simulink model "Assignment_2"  (R2022a)
settings: Solver=FixedStepAuto  StartTime=0.0  StopTime=10  FixedStep=1e-3  RelTol=1e-3  EnableMultiTasking=on
undefined symbols (not defined in the file or in its folder): D0, D1, D10, D11, D12, D13, D2, D3, D4, D5, D6, D7, D8, D9, PTA0, PTA1, PTA2, PTB23, PTB9, PTC16, PTC17, PTC2, PTC3, PTC4, PTD0, PTD1, PTD2, PTD3
libraries: etargetslib x25, frdmk64flib x16
settings Model: ExtModeTrigDuration=5  Creator=anand  LastModifiedBy=anand
settings DataIOCC: ReturnWorkspaceOutputs=off
settings OptimizationCC: EnhancedBackFolding=on  PassReuseOutputArgsAs=Individual arguments  ZeroExternalMemoryAtStartup=off  ZeroInternalMemoryAtStartup=off  MaxStackSize=64  OptimizeBlockOrder=speed  DifferentSizesBufferReuse=on  OptimizationCustomize=off  EfficientTunableParamExpr=on
settings DebuggingCC: ParameterTunabilityLossMsg=error
settings HardwareCC: ProdBitPerPointer=32  ProdBitPerSizeT=32  ProdBitPerPtrDiffT=32  ProdLargestAtomicInteger=Long  ProdLargestAtomicFloat=Double  ProdWordSize=32  ProdHWDeviceType=ARM Compatible->ARM Cortex
settings SFSimCC: MATLABDynamicMemAlloc=off
settings RTWCC: SystemTargetFile=ert.tlc  HardwareBoard=NXP FRDM-K64F  TLCOptions="-aInlineSetEventsForThisBaseRateFcn=TLC_FALSE -aSuppressMultiTaskScheduler=TLC_FALSE  -aRateBasedStepFcn=0"  TemplateMakefile=ert_default_tmf  Toolchain=GNU Tools for ARM Embedded Processors
settings CodeAppCC: ForceParamTrailComments=on  IgnoreCustomStorageClasses=off  OperatorAnnotations=on  SimulinkDataObjDesc=on  SFDataObjDesc=on  InsertBlockDesc=on
settings ERTTargetCC: ExtModeTransport=4  ExtModeMexFile=sendToCommService

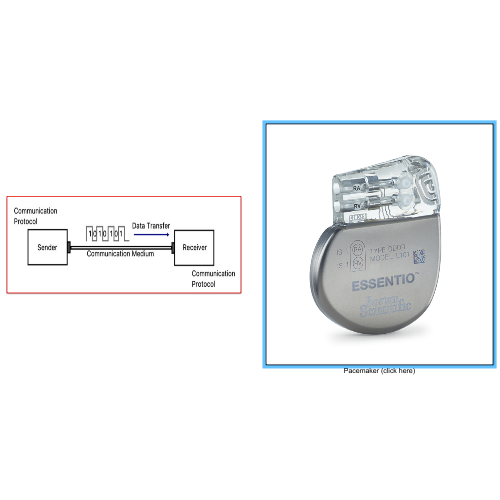
[thumbnail: Simulink's stored preview of the top-level diagram]
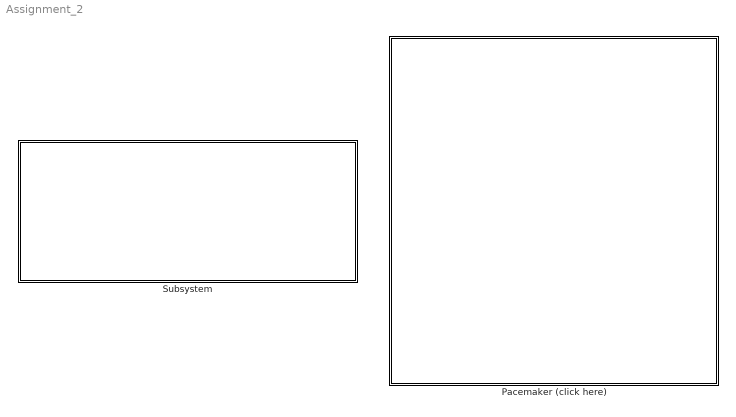
== system Assignment_2 ==
  Pacemaker (click here) : Subsystem
      mask Display: image('$imagefile'); % Use "Edit Image" on toolstrip to change.
  Subsystem : Subsystem
      mask Display: image('C:\Users\anand\Desktop\Screenshot 2022-11-24 140132.jpg'); % Use "Edit Image" on toolstrip to change.

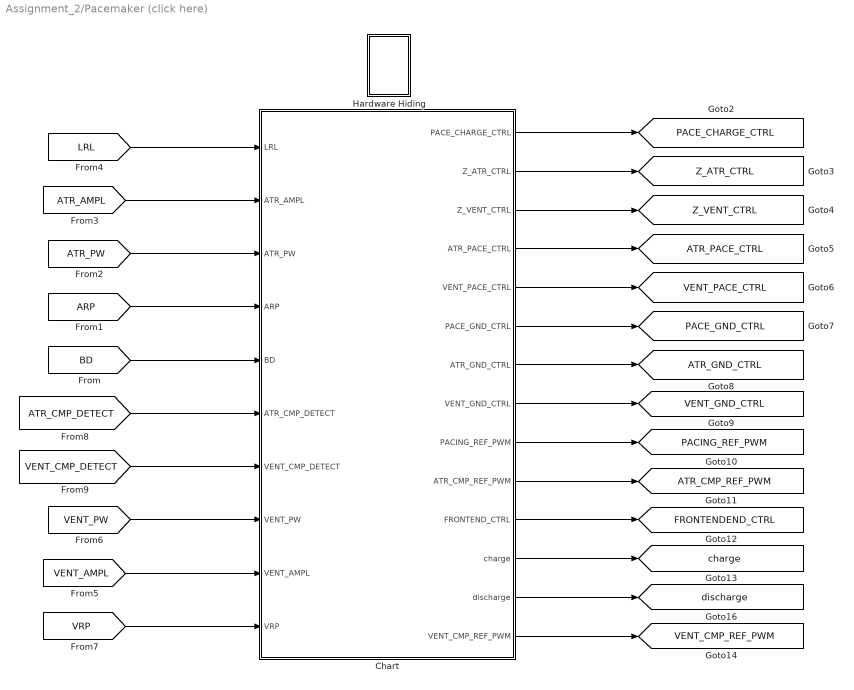
== system Assignment_2/Pacemaker (click here) ==
  Chart : Stateflow chart  TreatAsAtomicUnit=on
  Hardware Hiding : Subsystem
  tag scope: ATR_CMP_REF_PWM=global, ATR_GND_CTRL=global, ATR_PACE_CTRL=global, FRONTENDEND_CTRL=global, PACE_CHARGE_CTRL=global, PACE_GND_CTRL=global, PACING_REF_PWM=global, VENT_CMP_REF_PWM=global, VENT_GND_CTRL=global, VENT_PACE_CTRL=global, Z_ATR_CTRL=global, Z_VENT_CTRL=global, charge=global, discharge=global
  wires:
  Chart/9(PACING_REF_PWM) -> [PACING_REF_PWM]
  Chart/11(FRONTEND_CTRL) -> [FRONTENDEND_CTRL]
  Chart/10(ATR_CMP_REF_PWM) -> [ATR_CMP_REF_PWM]
  [ATR_CMP_DETECT] -> Chart/6(ATR_CMP_DETECT)
  [LRL] -> Chart/1(LRL)
  [VENT_AMPL] -> Chart/9(VENT_AMPL)
  Chart/4(ATR_PACE_CTRL) -> [ATR_PACE_CTRL]
  [ARP] -> Chart/4(ARP)
  [ATR_PW] -> Chart/3(ATR_PW)
  [BD] -> Chart/5(BD)
  Chart/14(VENT_CMP_REF_PWM) -> [VENT_CMP_REF_PWM]
  Chart/5(VENT_PACE_CTRL) -> [VENT_PACE_CTRL]
  Chart/12(charge) -> [charge]
  [ATR_AMPL] -> Chart/2(ATR_AMPL)
  Chart/6(PACE_GND_CTRL) -> [PACE_GND_CTRL]
  Chart/13(discharge) -> [discharge]
  Chart/2(Z_ATR_CTRL) -> [Z_ATR_CTRL]
  [VRP] -> Chart/10(VRP)
  Chart/3(Z_VENT_CTRL) -> [Z_VENT_CTRL]
  [VENT_CMP_DETECT] -> Chart/7(VENT_CMP_DETECT)
  Chart/7(ATR_GND_CTRL) -> [ATR_GND_CTRL]
  Chart/8(VENT_GND_CTRL) -> [VENT_GND_CTRL]
  Chart/1(PACE_CHARGE_CTRL) -> [PACE_CHARGE_CTRL]
  [VENT_PW] -> Chart/8(VENT_PW)

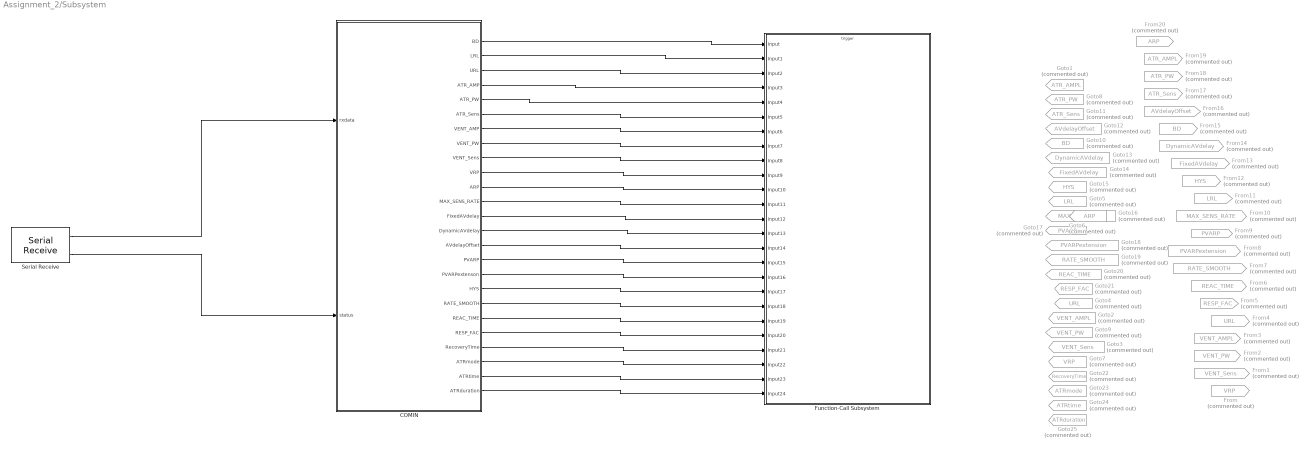
== system Assignment_2/Subsystem ==
  COMIN : Stateflow chart  TreatAsAtomicUnit=on
  From : From  Commented=on  GotoTag=VRP  TagVisibility=global
  From1 : From  Commented=on  GotoTag=VENT_Sens  TagVisibility=global
  From10 : From  Commented=on  GotoTag=MAX_SENS_RATE  TagVisibility=global
  From11 : From  Commented=on  GotoTag=LRL  TagVisibility=global
  From12 : From  Commented=on  GotoTag=HYS  TagVisibility=global
  From13 : From  Commented=on  GotoTag=FixedAVdelay  TagVisibility=global
  From14 : From  Commented=on  GotoTag=DynamicAVdelay  TagVisibility=global
  From15 : From  Commented=on  GotoTag=BD  TagVisibility=global
  From16 : From  Commented=on  GotoTag=AVdelayOffset  TagVisibility=global
  From17 : From  Commented=on  GotoTag=ATR_Sens  TagVisibility=global
  From18 : From  Commented=on  GotoTag=ATR_PW  TagVisibility=global
  From19 : From  Commented=on  GotoTag=ATR_AMPL  TagVisibility=global
  From2 : From  Commented=on  GotoTag=VENT_PW  TagVisibility=global
  From20 : From  Commented=on  GotoTag=ARP  TagVisibility=global
  From3 : From  Commented=on  GotoTag=VENT_AMPL  TagVisibility=global
  From4 : From  Commented=on  GotoTag=URL  TagVisibility=global
  From5 : From  Commented=on  GotoTag=RESP_FAC  TagVisibility=global
  From6 : From  Commented=on  GotoTag=REAC_TIME  TagVisibility=global
  From7 : From  Commented=on  GotoTag=RATE_SMOOTH  TagVisibility=global
  From8 : From  Commented=on  GotoTag=PVARPextension  TagVisibility=global
  From9 : From  Commented=on  GotoTag=PVARP  TagVisibility=global
  Function-Call Subsystem : Subsystem  TreatAsAtomicUnit=on
  Goto1 : Goto  Commented=on  GotoTag=ATR_AMPL  TagVisibility=global
  Goto10 : Goto  Commented=on  GotoTag=BD  TagVisibility=global
  Goto11 : Goto  Commented=on  GotoTag=ATR_Sens  TagVisibility=global
  Goto12 : Goto  Commented=on  GotoTag=AVdelayOffset  TagVisibility=global
  Goto13 : Goto  Commented=on  GotoTag=DynamicAVdelay  TagVisibility=global
  Goto14 : Goto  Commented=on  GotoTag=FixedAVdelay  TagVisibility=global
  Goto15 : Goto  Commented=on  GotoTag=HYS  TagVisibility=global
  Goto16 : Goto  Commented=on  GotoTag=MAX_SENS_RATE  TagVisibility=global
  Goto17 : Goto  Commented=on  GotoTag=PVARP  TagVisibility=global
  Goto18 : Goto  Commented=on  GotoTag=PVARPextension  TagVisibility=global
  Goto19 : Goto  Commented=on  GotoTag=RATE_SMOOTH  TagVisibility=global
  Goto2 : Goto  Commented=on  GotoTag=VENT_AMPL  TagVisibility=global
  Goto20 : Goto  Commented=on  GotoTag=REAC_TIME  TagVisibility=global
  Goto21 : Goto  Commented=on  GotoTag=RESP_FAC  TagVisibility=global
  Goto22 : Goto  Commented=on  GotoTag=RecoveryTime  TagVisibility=global
  Goto23 : Goto  Commented=on  GotoTag=ATRmode  TagVisibility=global
  Goto24 : Goto  Commented=on  GotoTag=ATRtime  TagVisibility=global
  Goto25 : Goto  Commented=on  GotoTag=ATRduration  TagVisibility=global
  Goto3 : Goto  Commented=on  GotoTag=VENT_Sens  TagVisibility=global
  Goto4 : Goto  Commented=on  GotoTag=URL  TagVisibility=global
  Goto5 : Goto  Commented=on  GotoTag=LRL  TagVisibility=global
  Goto6 : Goto  Commented=on  GotoTag=ARP  TagVisibility=global
  Goto7 : Goto  Commented=on  GotoTag=VRP  TagVisibility=global
  Goto8 : Goto  Commented=on  GotoTag=ATR_PW  TagVisibility=global
  Goto9 : Goto  Commented=on  GotoTag=VENT_PW  TagVisibility=global
  Serial Receive : frdmk64flib/Serial Receive  SCIModule=0  Baudrate=uint32(9600)  Parity=None  StopBits=1  HardwareFlowControl=None  ByteOrder=LittleEndian  DataType=uint8  DataLength=101  BlockingMode=off  OutputStatus=on  SampleTime=-1
  wires:
  Serial Receive/1 -> COMIN/1(rxdata)
  Serial Receive/2 -> COMIN/2(status)
  COMIN/1(BD) -> Function-Call Subsystem/1(Input)
  COMIN/2(LRL) -> Function-Call Subsystem/2(Input1)
  COMIN/3(URL) -> Function-Call Subsystem/3(Input2)
  COMIN/4(ATR_AMP) -> Function-Call Subsystem/4(Input3)
  COMIN/5(ATR_PW) -> Function-Call Subsystem/5(Input4)
  COMIN/6(ATR_Sens) -> Function-Call Subsystem/6(Input5)
  COMIN/7(VENT_AMP) -> Function-Call Subsystem/7(Input6)
  COMIN/8(VENT_PW) -> Function-Call Subsystem/8(Input7)
  COMIN/9(VENT_Sens) -> Function-Call Subsystem/9(Input8)
  COMIN/10(VRP) -> Function-Call Subsystem/10(Input9)
  COMIN/11(ARP) -> Function-Call Subsystem/11(Input10)
  COMIN/12(MAX_SENS_RATE) -> Function-Call Subsystem/12(Input11)
  COMIN/13(FixedAVdelay) -> Function-Call Subsystem/13(Input12)
  COMIN/14(DynamicAVdelay) -> Function-Call Subsystem/14(Input13)
  COMIN/15(AVdelayOffset) -> Function-Call Subsystem/15(Input14)
  COMIN/16(PVARP) -> Function-Call Subsystem/16(Input15)
  COMIN/17(PVARPextenson) -> Function-Call Subsystem/17(Input16)
  COMIN/18(HYS) -> Function-Call Subsystem/18(Input17)
  COMIN/19(RATE_SMOOTH) -> Function-Call Subsystem/19(Input18)
  COMIN/20(REAC_TIME) -> Function-Call Subsystem/20(Input19)
  COMIN/21(RESP_FAC) -> Function-Call Subsystem/21(Input20)
  COMIN/22(RecoveryTime) -> Function-Call Subsystem/22(Input21)
  COMIN/23(ATRmode) -> Function-Call Subsystem/23(Input22)
  COMIN/24(ATRtime) -> Function-Call Subsystem/24(Input23)
  COMIN/25(ATRduration) -> Function-Call Subsystem/25(Input24)

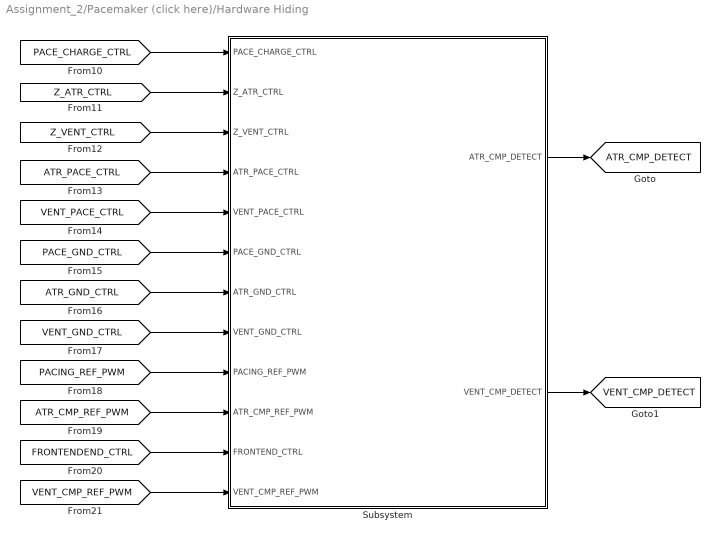
== system Assignment_2/Pacemaker (click here)/Hardware Hiding ==
  Subsystem : Subsystem
  tag scope: ATR_CMP_DETECT=global, VENT_CMP_DETECT=global
  wires:
  [PACE_GND_CTRL] -> Subsystem/6(PACE_GND_CTRL)
  Subsystem/1(ATR_CMP_DETECT) -> [ATR_CMP_DETECT]
  [Z_ATR_CTRL] -> Subsystem/2(Z_ATR_CTRL)
  [FRONTENDEND_CTRL] -> Subsystem/11(FRONTEND_CTRL)
  [ATR_CMP_REF_PWM] -> Subsystem/10(ATR_CMP_REF_PWM)
  [Z_VENT_CTRL] -> Subsystem/3(Z_VENT_CTRL)
  Subsystem/2(VENT_CMP_DETECT) -> [VENT_CMP_DETECT]
  [PACE_CHARGE_CTRL] -> Subsystem/1(PACE_CHARGE_CTRL)
  [VENT_GND_CTRL] -> Subsystem/8(VENT_GND_CTRL)
  [ATR_GND_CTRL] -> Subsystem/7(ATR_GND_CTRL)
  [PACING_REF_PWM] -> Subsystem/9(PACING_REF_PWM)
  [VENT_PACE_CTRL] -> Subsystem/5(VENT_PACE_CTRL)
  [ATR_PACE_CTRL] -> Subsystem/4(ATR_PACE_CTRL)
  [VENT_CMP_REF_PWM] -> Subsystem/12(VENT_CMP_REF_PWM)

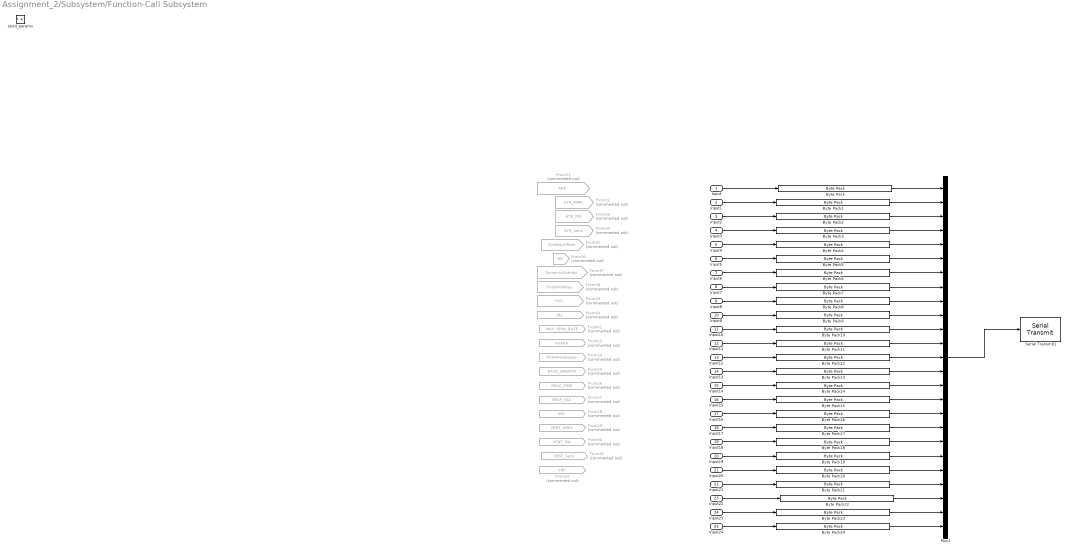
== system Assignment_2/Subsystem/Function-Call Subsystem ==
  Input : Inport  OutDataTypeStr=int32
  Input1 : Inport  Port=2
  Input2 : Inport  Port=3
  Input3 : Inport  Port=4
  Input4 : Inport  Port=5
  Input5 : Inport  Port=6
  Input6 : Inport  Port=7
  Input7 : Inport  Port=8
  Input8 : Inport  Port=9
  Input9 : Inport  Port=10
  Input10 : Inport  Port=11
  Input11 : Inport  Port=12
  Input12 : Inport  Port=13
  Input13 : Inport  Port=14
  Input14 : Inport  Port=15
  Input15 : Inport  Port=16
  Input16 : Inport  Port=17
  Input17 : Inport  Port=18
  Input18 : Inport  Port=19
  Input19 : Inport  Port=20
  Input20 : Inport  Port=21
  Input21 : Inport  Port=22
  Input22 : Inport  Port=23
  Input23 : Inport  Port=24
  Input24 : Inport  Port=25
  send_params : TriggerPort  TriggerType=function-call  IsSimulinkFunction=on  FunctionName=send_params  VariantControl=(inherit)
  Byte Pack{,1..2,9..24} (19 alike) : etargetslib/Byte Pack  datatypes={'int32'}  byteAlign=1
  Byte Pack{3..8} (6 alike) : etargetslib/Byte Pack  datatypes={'single'}  byteAlign=1
  From21 : From  Commented=on  GotoTag=ARP  TagVisibility=global
  From22 : From  Commented=on  GotoTag=ATR_AMPL  TagVisibility=global
  From23 : From  Commented=on  GotoTag=PVARP  TagVisibility=global
  From24 : From  Commented=on  GotoTag=PVARPextension  TagVisibility=global
  From25 : From  Commented=on  GotoTag=RATE_SMOOTH  TagVisibility=global
  From26 : From  Commented=on  GotoTag=REAC_TIME  TagVisibility=global
  From27 : From  Commented=on  GotoTag=RESP_FAC  TagVisibility=global
  From28 : From  Commented=on  GotoTag=URL  TagVisibility=global
  From29 : From  Commented=on  GotoTag=VENT_AMPL  TagVisibility=global
  From30 : From  Commented=on  GotoTag=VENT_PW  TagVisibility=global
  From31 : From  Commented=on  GotoTag=VENT_Sens  TagVisibility=global
  From32 : From  Commented=on  GotoTag=VRP  TagVisibility=global
  From33 : From  Commented=on  GotoTag=ATR_PW  TagVisibility=global
  From34 : From  Commented=on  GotoTag=ATR_Sens  TagVisibility=global
  From35 : From  Commented=on  GotoTag=AVdelayOffset  TagVisibility=global
  From36 : From  Commented=on  GotoTag=BD  TagVisibility=global
  From37 : From  Commented=on  GotoTag=DynamicAVdelay  TagVisibility=global
  From38 : From  Commented=on  GotoTag=FixedAVdelay  TagVisibility=global
  From39 : From  Commented=on  GotoTag=HYS  TagVisibility=global
  From40 : From  Commented=on  GotoTag=LRL  TagVisibility=global
  From41 : From  Commented=on  GotoTag=MAX_SENS_RATE  TagVisibility=global
  Mux1 : Mux  Inputs=25
  Serial Transmit1 : frdmk64flib/Serial Transmit  SCIModule=0  Baudrate=uint32(9600)  Parity=None  StopBits=1  HardwareFlowControl=None  ByteOrder=LittleEndian  BlockingMode=on  OutputStatus=off
  wires:
  Mux1/1 -> Serial Transmit1/1
  Input/1 -> Byte Pack/1
  Byte Pack/1 -> Mux1/1
  Byte Pack1/1 -> Mux1/2
  Byte Pack2/1 -> Mux1/3
  Input1/1 -> Byte Pack1/1
  Input2/1 -> Byte Pack2/1
  Byte Pack3/1 -> Mux1/4
  Byte Pack4/1 -> Mux1/5
  Byte Pack5/1 -> Mux1/6
  Byte Pack6/1 -> Mux1/7
  Byte Pack7/1 -> Mux1/8
  Byte Pack8/1 -> Mux1/9
  Byte Pack9/1 -> Mux1/10
  Byte Pack10/1 -> Mux1/11
  Byte Pack11/1 -> Mux1/12
  Byte Pack12/1 -> Mux1/13
  Byte Pack13/1 -> Mux1/14
  Byte Pack14/1 -> Mux1/15
  Byte Pack15/1 -> Mux1/16
  Byte Pack16/1 -> Mux1/17
  Byte Pack17/1 -> Mux1/18
  Byte Pack18/1 -> Mux1/19
  Byte Pack19/1 -> Mux1/20
  Byte Pack20/1 -> Mux1/21
  Input3/1 -> Byte Pack3/1
  Input4/1 -> Byte Pack4/1
  Input5/1 -> Byte Pack5/1
  Input6/1 -> Byte Pack6/1
  Input7/1 -> Byte Pack7/1
  Input8/1 -> Byte Pack8/1
  Input9/1 -> Byte Pack9/1
  Input10/1 -> Byte Pack10/1
  Input11/1 -> Byte Pack11/1
  Input12/1 -> Byte Pack12/1
  Input13/1 -> Byte Pack13/1
  Input14/1 -> Byte Pack14/1
  Input15/1 -> Byte Pack15/1
  Input16/1 -> Byte Pack16/1
  Input17/1 -> Byte Pack17/1
  Input18/1 -> Byte Pack18/1
  Input19/1 -> Byte Pack19/1
  Input20/1 -> Byte Pack20/1
  Input21/1 -> Byte Pack21/1
  Input22/1 -> Byte Pack22/1
  Input23/1 -> Byte Pack23/1
  Input24/1 -> Byte Pack24/1
  Byte Pack21/1 -> Mux1/22
  Byte Pack22/1 -> Mux1/23
  Byte Pack23/1 -> Mux1/24
  Byte Pack24/1 -> Mux1/25

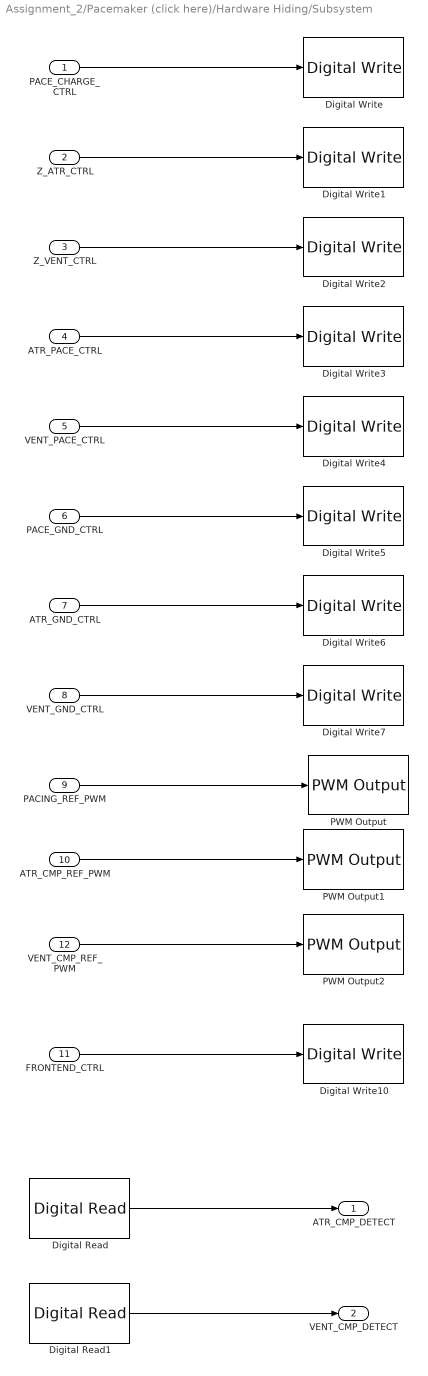
== system Assignment_2/Pacemaker (click here)/Hardware Hiding/Subsystem ==
  PACE_CHARGE_CTRL : Inport  OutDataTypeStr=boolean
  Z_ATR_CTRL : Inport  Port=2  OutDataTypeStr=boolean
  Z_VENT_CTRL : Inport  Port=3
  ATR_PACE_CTRL : Inport  Port=4
  VENT_PACE_CTRL : Inport  Port=5
  PACE_GND_CTRL : Inport  Port=6
  ATR_GND_CTRL : Inport  Port=7
  VENT_GND_CTRL : Inport  Port=8
  PACING_REF_PWM : Inport  Port=9
  ATR_CMP_REF_PWM : Inport  Port=10
  FRONTEND_CTRL : Inport  Port=11
  VENT_CMP_REF_PWM : Inport  Port=12
  Digital Read : frdmk64flib/Digital Read  Whichpin=PTC16 (D0)  SampleTime=-1
  Digital Read1 : frdmk64flib/Digital Read  Whichpin=PTC17 (D1)  SampleTime=-1
  Digital Write : frdmk64flib/Digital Write  Whichpin=PTB9 (D2)
  Digital Write1 : frdmk64flib/Digital Write  Whichpin=PTB23 (D4)
  Digital Write10 : frdmk64flib/Digital Write  Whichpin=PTD1 (D13)
  Digital Write2 : frdmk64flib/Digital Write  Whichpin=PTC3 (D7)
  Digital Write3 : frdmk64flib/Digital Write  Whichpin=PTA0 (D8)
  Digital Write4 : frdmk64flib/Digital Write  Whichpin=PTC4 (D9)
  Digital Write5 : frdmk64flib/Digital Write  Whichpin=PTD0 (D10)
  Digital Write6 : frdmk64flib/Digital Write  Whichpin=PTD2 (D11)
  Digital Write7 : frdmk64flib/Digital Write  Whichpin=PTD3 (D12)
  PWM Output : frdmk64flib/PWM Output  Whichpin=PTA2 (D5)  InitialFrequency=2000  InitialDutyCycle=0
  PWM Output1 : frdmk64flib/PWM Output  Whichpin=PTC2 (D6)  InitialFrequency=2000  InitialDutyCycle=0
  PWM Output2 : frdmk64flib/PWM Output  Whichpin=PTA1 (D3)  InitialFrequency=2000  InitialDutyCycle=0
  ATR_CMP_DETECT : Outport  OutDataTypeStr=boolean
  VENT_CMP_DETECT : Outport  Port=2  OutDataTypeStr=boolean
  wires:
  PACE_CHARGE_CTRL/1 -> Digital Write/1
  Z_ATR_CTRL/1 -> Digital Write1/1
  Z_VENT_CTRL/1 -> Digital Write2/1
  ATR_PACE_CTRL/1 -> Digital Write3/1
  VENT_PACE_CTRL/1 -> Digital Write4/1
  PACE_GND_CTRL/1 -> Digital Write5/1
  ATR_GND_CTRL/1 -> Digital Write6/1
  VENT_GND_CTRL/1 -> Digital Write7/1
  PACING_REF_PWM/1 -> PWM Output/1
  ATR_CMP_REF_PWM/1 -> PWM Output1/1
  Digital Read/1 -> ATR_CMP_DETECT/1
  FRONTEND_CTRL/1 -> Digital Write10/1
  Digital Read1/1 -> VENT_CMP_DETECT/1
  VENT_CMP_REF_PWM/1 -> PWM Output2/1

== stateflow chart Assignment_2/Subsystem/COMIN ==
  state SET_PARAM
    entry:
    BD = typecast(rxdata(3:6),'int32');
    LRL = typecast(rxdata(7:10),'int32');
    URL = typecast(rxdata(11:14),'int32');
    ATR_AMP = typecast(rxdata(15:18),'single');
    ATR_PW = typecast(rxdata(19:22),'single');
    ATR_Sens = typecast(rxdata(23:26),'single');
    VENT_AMP = typecast(rxdata(27:30),'single');
    VENT_PW = typecast(rxdata(31:34),'single');
    VENT_Sens = typecast(rxdata(35:38),'single');
    VRP = typecast(rxdata(39:42),'int32');
    ARP = typecast(rxdata(43:46),'int32');
    MAX_SENS_RATE = typecast(rxdata(47:50),'int32');
    FixedAVdelay = typecast(rxdata(51:54),'int32');
    DynamicAVdelay = typecast(rxdata(55:58),'int32');
    AVdelayOffset = typecast(rxdata(59:62),'int32');
    PVARP = typecast(rxdata(63:66),'int32');
    PVARPextenson = typecast(rxdata(67:70),'int32');
    HYS = typecast(rxdata(71:74),'int32');
    RATE_SMOOTH = typecast(rxdata(75:78),'int32');
    REAC_TIME = typecast(rxdata(79:82),'int32');
    RESP_FAC= typecast(rxdata(83:86),'int32');
    RecoveryTime = typecast(rxdata(87:90),'int32');
    ATRmode =  typecast(rxdata(91:94),'int32');
    ATRtime =  typecast(rxdata(94:97),'int32');
    ATRduration =  typecast(rxdata(98:101),'int32');
  state Initial
    entry:
  state STANDBY
  state ECHO_PARAM
    entry:
    send_params();
  (default) -> Initial
  SET_PARAM -> STANDBY
  (junction 9) -> STANDBY [order 2]
  (junction 6) -> SET_PARAM [order 1] : [rxdata(2) == hex2dec ('55')]
  Initial -> STANDBY
  STANDBY -> (junction 9) : [status==0]
  (junction 9) -> (junction 6) [order 1] : [rxdata(1) == hex2dec ('16')]
  (junction 6) -> ECHO_PARAM [order 2] : [rxdata(2) == hex2dec ('22')]
  ECHO_PARAM -> STANDBY
  data: BD output int32; LRL output int32; URL output int32; ATR_AMP output single; ATR_PW output single; ATR_Sens output single; VENT_AMP output single; VENT_PW output single; VENT_Sens output single; VRP output int32; rxdata input uint8; status input uint8; ARP output int32; MAX_SENS_RATE output int32; FixedAVdelay output int32; DynamicAVdelay output int32; AVdelayOffset output int32; PVARP output int32; PVARPextenson output int32; HYS output int32; RATE_SMOOTH output int32; REAC_TIME output int32; RESP_FAC output int32; RecoveryTime output int32; ATRmode output int32; ATRtime output int32; ATRduration output int32

== stateflow chart Assignment_2/Pacemaker (click here)/Chart ==
  state AOO
    state CHARGING_DISCHARGING
      entry:
      charge = true;
      %DISCHARGING C21
      PACE_GND_CTRL = true;
      VENT_PACE_CTRL = false;
      Z_ATR_CTRL = false;
      Z_VENT_CTRL = false;
      ATR_PACE_CTRL = false;
      ATR_GND_CTRL = true;
      VENT_GND_CTRL = false;
      %CHARGING C22
      PACING_REF_PWM = 100*ATR_AMPL/5;
      PACE_CHARGE_CTRL = true;
    state PACE_ATR
      entry:
      charge = false;
      PACE_CHARGE_CTRL = false;
      PACE_GND_CTRL = true;
      ATR_PACE_CTRL = true;
      ATR_GND_CTRL = false;
      Z_ATR_CTRL = false;
      Z_VENT_CTRL = false;
      VENT_GND_CTRL = false;
      VENT_PACE_CTRL = false;
    (default) -> AOO.CHARGING_DISCHARGING
    AOO.CHARGING_DISCHARGING -> AOO.PACE_ATR : [after(60000/LRL-ATR_PW, msec)]
    AOO.PACE_ATR -> AOO.CHARGING_DISCHARGING : [after(ATR_PW,msec)]
  state VOO
    state CHARGING_DISCHARGING
      entry:
      charge = true;
      %DISCHARGING C21
      PACE_GND_CTRL = true;
      VENT_PACE_CTRL = false;
      Z_ATR_CTRL = false;
      Z_VENT_CTRL = false;
      ATR_PACE_CTRL = false;
      ATR_GND_CTRL = true;
      VENT_GND_CTRL = false;
      %CHARGING C22
      PACING_REF_PWM = 100*VENT_AMPL/5;
      PACE_CHARGE_CTRL = true;
    state PACE_ATR
      entry:
      charge = false;
      PACE_CHARGE_CTRL = false;
      PACE_GND_CTRL = true;
      ATR_PACE_CTRL = false;
      ATR_GND_CTRL = false;
      Z_ATR_CTRL = false;
      Z_VENT_CTRL = false;
      VENT_GND_CTRL = false;
      VENT_PACE_CTRL = true;
    (default) -> VOO.CHARGING_DISCHARGING
    VOO.CHARGING_DISCHARGING -> VOO.PACE_ATR : [after(60000/LRL-VENT_PW, msec)]
    VOO.PACE_ATR -> VOO.CHARGING_DISCHARGING : [after(VENT_PW,msec)]
  state Start
    entry:
  state AAI
    state CHARGING
      entry:
      %CHARGING C22
      charge = true;
      discharge = false;
      FRONTEND_CTRL = true;
      VENT_PACE_CTRL = false;
      ATR_PACE_CTRL = false;
      PACING_REF_PWM = 90;
      PACE_CHARGE_CTRL = true;
      ATR_CMP_REF_PWM = 75;
    state PACE_ATR
      entry:
      charge = false;
      discharge = false;
      PACE_CHARGE_CTRL = false;
      PACE_GND_CTRL = true;
      VENT_PACE_CTRL = false;
      VENT_GND_CTRL = false;
      Z_VENT_CTRL = false;
      Z_ATR_CTRL = false;
      ATR_GND_CTRL = false;
      ATR_PACE_CTRL = true;
    state Atrial_Refractory_Period_Post_Sensing
    state DISCHARGING
      entry:
      %DISCHARGING C21
      charge = false;
      discharge = true;
      PACE_GND_CTRL = true;
      ATR_PACE_CTRL = false;
      Z_VENT_CTRL = false;
      Z_ATR_CTRL = false;
      VENT_PACE_CTRL = false;
      VENT_GND_CTRL = false;
      ATR_GND_CTRL = true;
    (default) -> AAI.CHARGING : {delta =  0; sensing = 0}
    AAI.CHARGING -> Atrial_Refractory_Period_Post_Sensing [order 1] : [ATR_CMP_DETECT == true]
    AAI.CHARGING -> AAI.PACE_ATR [order 2] : [after(60000/LRL-delta-ATR_PW, msec)]
    Atrial_Refractory_Period_Post_Sensing -> AAI.CHARGING : [after(ARP+35,msec)]{delta = ARP; sensing = 1}
    (junction 210) -> AAI.CHARGING : [after(1, msec)]{delta = 0; sensing = 0}
    (junction 198) -> AAI.CHARGING : [after(ARP,msec)]{delta = ARP}
    AAI.PACE_ATR -> AAI.DISCHARGING : [after(ATR_PW,msec)]
    AAI.DISCHARGING -> (junction 198) [order 1] : [sensing == 0]
    AAI.DISCHARGING -> (junction 210) [order 2] : [sensing == 1]
  state VVI
    state CHARGING
      entry:
      %CHARGING C22
      FRONTEND_CTRL = true;
      ATR_PACE_CTRL = false;
      VENT_PACE_CTRL = false;
      PACING_REF_PWM = 90;
      PACE_CHARGE_CTRL = true;
      VENT_CMP_REF_PWM = 75;
    state PACE_ATR
      entry:
      PACE_CHARGE_CTRL = false;
      PACE_GND_CTRL = true;
      ATR_PACE_CTRL = false;
      ATR_GND_CTRL = false;
      Z_ATR_CTRL = false;
      Z_VENT_CTRL = false;
      VENT_GND_CTRL = false;
      VENT_PACE_CTRL = true;
    state Ventricular_Refractory_Period_Post_Sensing
    state DISCHARGING
      entry:
      %DISCHARGING C21
      PACE_GND_CTRL = true;
      VENT_PACE_CTRL = false;
      Z_ATR_CTRL = false;
      Z_VENT_CTRL = false;
      ATR_PACE_CTRL = false;
      ATR_GND_CTRL = false;
      VENT_GND_CTRL = true;
    (default) -> VVI.CHARGING : {delta = 0; sensing = 0}
    VVI.CHARGING -> Ventricular_Refractory_Period_Post_Sensing [order 1] : [VENT_CMP_DETECT == true]
    VVI.CHARGING -> VVI.PACE_ATR [order 2] : [after(60000/LRL-delta-VENT_PW, msec)]
    Ventricular_Refractory_Period_Post_Sensing -> VVI.CHARGING : [after(VRP+35,msec)]{delta = VRP; sensing = 1}
    (junction 215) -> VVI.CHARGING : [after(1, msec)]{delta = 0; sensing = 0}
    (junction 214) -> VVI.CHARGING : [after(VRP,msec)]{delta = VRP}
    VVI.PACE_ATR -> VVI.DISCHARGING : [after(VENT_PW,msec)]
    VVI.DISCHARGING -> (junction 214) [order 1] : [sensing == 0]
    VVI.DISCHARGING -> (junction 215) [order 2] : [sensing == 1]
  Start -> AOO [order 1] : [BD == 1]
  Start -> VOO [order 2] : [BD == 2]
  (default) -> Start
  Start -> AAI [order 3] : [BD == 3]
  Start -> VVI [order 4] : [BD == 4]
  data: LRL input single; ATR_AMPL input single; ATR_PW input single; PACE_CHARGE_CTRL output boolean; Z_ATR_CTRL output; Z_VENT_CTRL output; ATR_PACE_CTRL output; VENT_PACE_CTRL output; PACE_GND_CTRL output; ATR_GND_CTRL output; VENT_GND_CTRL output; PACING_REF_PWM output single; ARP input single; ATR_CMP_REF_PWM output; delta local single; FRONTEND_CTRL output boolean; BD input; ATR_CMP_DETECT input boolean size=[1,1]; VENT_CMP_DETECT input boolean size=[1,1]; sensing local; VENT_PW input; VENT_AMPL input single; charge output boolean; discharge output boolean; VENT_CMP_REF_PWM output; VRP input single
